simulink model "motor_model"  (R2025b)
settings: Solver=VariableStepAuto  StartTime=0.0  StopTime=10.0  RelTol=1e-3
values from neighbouring files (symbols this model uses):
  b = 3.5077e-6    (= 3.5077e-06)    [load_parameters.m]
  J = 3.2284e-6    (= 3.2284e-06)    [load_parameters.m]
  K = 0.0274    [load_parameters.m]
  L = 2.75e-6    (= 2.75e-06)    [load_parameters.m]
  R = 4    [load_parameters.m]
settings Model: Creator=REARDONNM24  LastModifiedBy=REARDONNM24

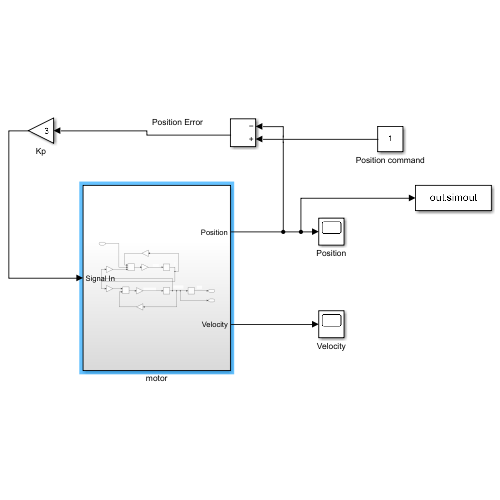
[thumbnail: Simulink's stored preview of the top-level diagram]
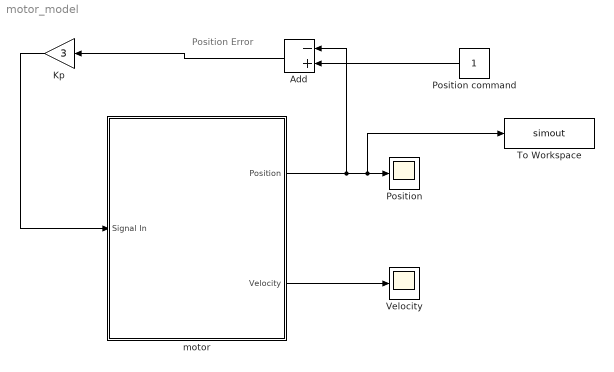
== system motor_model ==
  note: Position Error
  Add : Sum  Inputs=-+
  Kp : Gain  Gain=3
  Position : Scope
      settings: ActiveDisplayYMinimum=0.90254200315002775  ActiveDisplayYMaximum=1.0689345783117008
  Position command : Constant
  To Workspace : ToWorkspace  VariableName=simout  SaveFormat=Timeseries  SampleTime=-1
  Velocity : Scope
      settings: ActiveDisplayYMinimum=174.41543511722466  ActiveDisplayYMaximum=4357.1108128089754
  motor : Subsystem
  wires:
  motor/1(Position) -> Add/1, To Workspace/1, Position/1
  motor/2(Velocity) -> Velocity/1
  Add/1 -> Kp/1
  Kp/1 -> motor/1(Signal In)
  Position command/1 -> Add/2

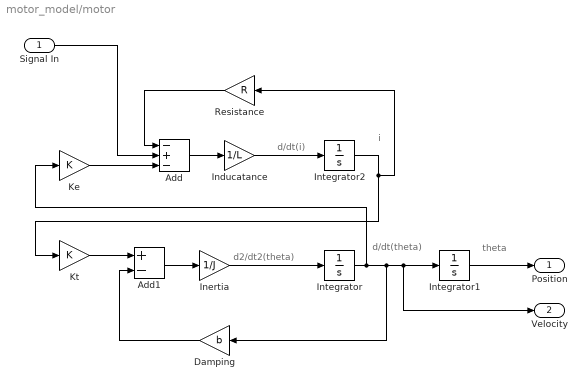
== system motor_model/motor ==
  note: i
  note: d/dt(i)
  note: theta
  note: d/dt(theta)
  note: d2/dt2(theta)
  Signal In : Inport
  Add : Sum  Inputs=-+-
  Add1 : Sum  Inputs=+-
  Damping : Gain  Gain=b
  Inducatance : Gain  Gain=1/L
  Inertia : Gain  Gain=1/J
  Integrator : Integrator
  Integrator1 : Integrator
  Integrator2 : Integrator
  Ke : Gain  Gain=K
  Kt : Gain  Gain=K
  Resistance : Gain  Gain=R
  Position : Outport
  Velocity : Outport  Port=2
  wires:
  Signal In/1 -> Add/2
  Resistance/1 -> Add/1
  Inertia/1 -> Integrator/1
  Integrator/1 -> Ke/1, Damping/1, Velocity/1, Integrator1/1
  Integrator2/1 -> Resistance/1, Kt/1
  Damping/1 -> Add1/2
  Inducatance/1 -> Integrator2/1
  Add1/1 -> Inertia/1
  Add/1 -> Inducatance/1
  Kt/1 -> Add1/1
  Ke/1 -> Add/3
  Integrator1/1 -> Position/1
